simulink model "PCM_Encoder_Decoder"  (R2024b)
settings: Solver=VariableStepAuto  StartTime=0.0  StopTime=10.0  RelTol=1e-3
libraries: simulink x2, dspquant2 x2, dspfdesign x1, dspsigops x1
settings Model: Creator=white  LastModifiedBy=white

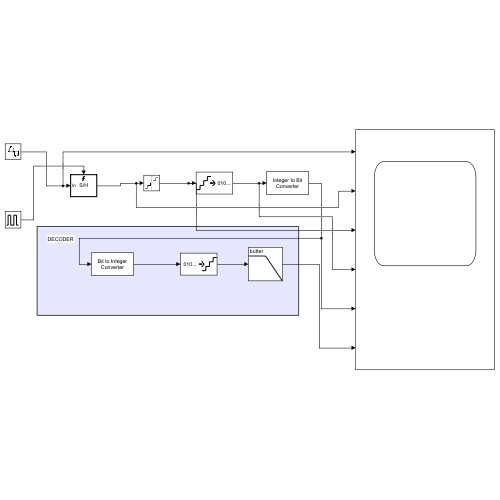
[thumbnail: Simulink's stored preview of the top-level diagram]
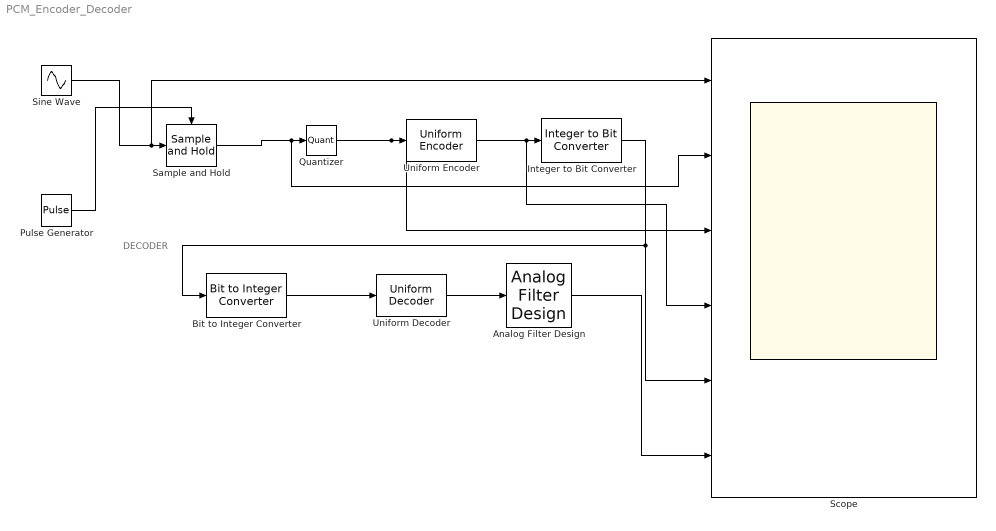
== system PCM_Encoder_Decoder ==
  note: DECODER
  Analog Filter Design : dspfdesign/Analog Filter Design  method=Butterworth  filttype=Lowpass  N=8  Wlo=2*pi*2  Whi=80  Rp=2  Rs=40
  Bit to Integer Converter : simulink/Logic and Bit Operations/Bit to Integer Converter  nbits=2  bitOrder=MSB first  signedOutputValues=Signed  outDtype=Inherit via internal rule  outDtypeSigned=Inherit via internal rule
  Integer to Bit Converter : simulink/Logic and Bit Operations/Integer to Bit Converter  nbits=2  signedInputValues=Signed  bitOrder=MSB first  outDtype=Inherit via internal rule
  Pulse Generator : DiscretePulseGenerator  PulseType=Time based  Amplitude=10  Period=1/40  PulseWidth=5
  Quantizer : Quantizer  QuantizationInterval=5
  Sample and Hold : dspsigops/Sample and Hold  trig=Rising edge  initCond=0  latchinput=off
  Scope : Scope  NumInputPorts=6
  Sine Wave : Sin  Amplitude=10  Frequency=2*pi*2  SampleTime=1/10000
  Uniform Decoder : dspquant2/Uniform Decoder  peak=1  bits=2  overflowMode=Saturate  otype=double
  Uniform Encoder : dspquant2/Uniform Encoder  peak=1  bits=2  otype=Signed integer
  wires:
  Sine Wave/1 -> Scope/1, Sample and Hold/1
  Pulse Generator/1 -> Sample and Hold/Trigger
  Sample and Hold/1 -> Scope/2, Quantizer/1
  Quantizer/1 -> Scope/3, Uniform Encoder/1
  Uniform Encoder/1 -> Scope/4, Integer to Bit Converter/1
  Integer to Bit Converter/1 -> Scope/5, Bit to Integer Converter/1
  Bit to Integer Converter/1 -> Uniform Decoder/1
  Uniform Decoder/1 -> Analog Filter Design/1
  Analog Filter Design/1 -> Scope/6
